simulink model "DJI_Mavic_Pro"  (R2022b)
settings: Solver=VariableStepAuto  StartTime=0.0  StopTime=100  RelTol=1e-3
libraries: slpidlib x3
settings Model: Creator=vikram  LastModifiedBy=vikram

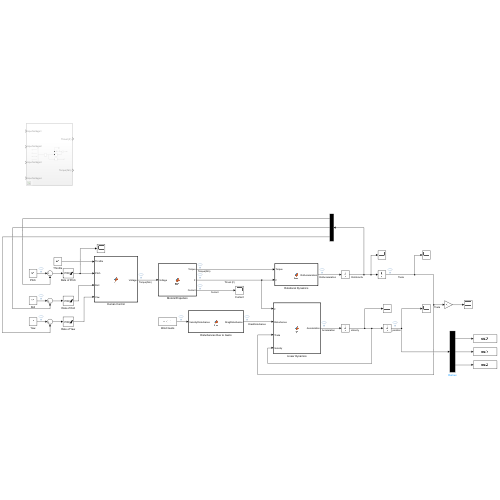
[thumbnail: Simulink's stored preview of the top-level diagram]
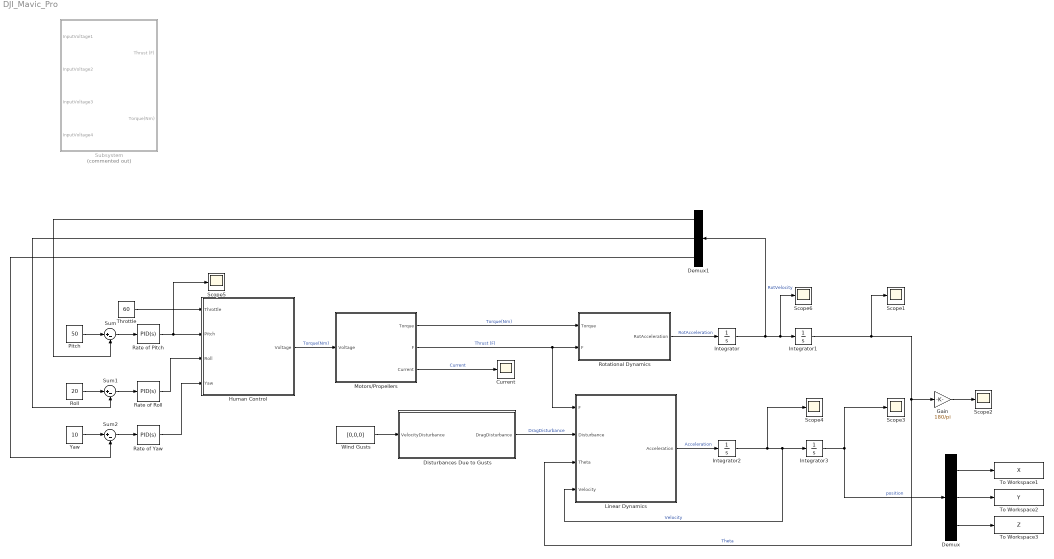
== system DJI_Mavic_Pro ==
  Current : Scope
  Demux : Demux  Outputs=3
  Demux1 : Demux  Outputs=3
  Disturbances Due to Gusts : MATLAB Function  TreatAsAtomicUnit=on
  Gain : Gain  Gain=180/pi
  Human Control : MATLAB Function  TreatAsAtomicUnit=on
  Integrator{,1..3} (4 alike) : Integrator
  Linear Dynamics : MATLAB Function  TreatAsAtomicUnit=on
  Motors/Propellers : MATLAB Function  TreatAsAtomicUnit=on
  Pitch : Constant  Value=50
  Rate of Pitch : slpidlib/PID Controller  Controller=PID  Form=Parallel  TimeDomain=Continuous-time  UseExternalTs=off  SampleTime=-1  IntegratorMethod=Forward Euler  FilterMethod=Forward Euler  ControllerParametersSource=internal  P=10  I=5  UseKiTs=off  D=0  N=100  UseFilter=on  TunerSelectOption=Transfer Function Based (PID Tuner App)  InitialConditionSource=internal  InitialConditionForIntegrator=0  InitialConditionForFilter=0  DifferentiatorICPrevScaledInput=0  ExternalReset=none  TrackingMode=off  Kt=1  LimitOutput=on  SatLimitsSource=internal  UpperSaturationLimit=100  LowerSaturationLimit=0  LinearizeAsGain=on  AntiWindupMode=clamping  Kb=1  LimitIntegrator=off  UpperIntegratorSaturationLimit=inf  LowerIntegratorSaturationLimit=-inf  POutMin=[]  POutMax=[]  IOutMin=[]  IOutMax=[]  DOutMin=[]  DOutMax=[]  NOutMin=[]  NOutMax=[]  SumOutMin=[]  SumOutMax=[]  SaturationOutMin=[]  SaturationOutMax=[]  PParamMin=[]  PParamMax=[]  IParamMin=[]  IParamMax=[]  DParamMin=[]  DParamMax=[]  NParamMin=[]  NParamMax=[]  KbParamMin=[]  KbParamMax=[]  KtParamMin=[]  KtParamMax=[]  KbOutMin=[]  KbOutMax=[]  KtOutMin=[]  KtOutMax=[]  IntegratorOutMin=[]  IntegratorOutMax=[]  FilterOutMin=[]  FilterOutMax=[]  SumI1OutMin=[]  SumI1OutMax=[]  SumI2OutMin=[]  SumI2OutMax=[]  SumI3OutMin=[]  SumI3OutMax=[]  SumI4OutMin=[]  SumI4OutMax=[]  SumDOutMin=[]  SumDOutMax=[]  DifferentiatorOutMin=[]  DifferentiatorOutMax=[]  FilterDiffOutCoefMin=[]  FilterDiffOutCoefMax=[]  ReciprocalOutMin=[]  ReciprocalOutMax=[]  SumDenOutMin=[]  SumDenOutMax=[]  SumNumOutMin=[]  SumNumOutMax=[]  DivideOutMin=[]  DivideOutMax=[]  UdiffTsProdOutMin=[]  UdiffTsProdOutMax=[]  NTsProdOutMin=[]  NTsProdOutMax=[]  UintegralTsProdOutMin=[]  UintegralTsProdOutMax=[]  UngainTsProdOutMin=[]  UngainTsProdOutMax=[]  ClampingZeroOutDataTypeStr=Inherit: Inherit via back propagation  ClampingZeroOutMin=[]  ClampingZeroOutMax=[]  FilterDenConstantOutDataTypeStr=Inherit: Inherit via back propagation  FilterDenConstantOutMin=[]  FilterDenConstantOutMax=[]  PCopyOutDataTypeStr=Inherit: Inherit via back propagation  PCopyOutMin=[]  PCopyOutMax=[]  NCopyOutDataTypeStr=Inherit: Inherit via back propagation  NCopyOutMin=[]  NCopyOutMax=[]  IntegratorContinuousStateAttributes=''  IntegratorStateMustResolveToSignalObject=off  IntegratorRTWStateStorageClass=Auto  FilterContinuousStateAttributes=''  FilterStateMustResolveToSignalObject=off  FilterRTWStateStorageClass=Auto  ParallelPVariant=InternalParameters  IdealPVariant=Disabled  IVariant=InternalParameters  DVariant=InternalParameters  IntegratorVariant=Continuous  SatVariant=Enabled  AWVariant=ContClampingParallel  PCopyVariant=Disabled  TRVariant=Disabled  FdbkBlocksVariant=Forward  IdealPFdbkVariant=Disabled  SatFdbkVariant=Disabled  DerivativeFilterVariant=ContFilter  NVariant=InternalParameters  NCopyVariant=Disabled  FilterICVariant=InternalICsFilter  IntegratorICVariant=InternalICs  ExternalResetVariant=Disabled  TRSumVariant=Passthrough  SumFdbkVariant=Disabled  SumVariant=Sum_PID  TsampFilterVariant=InternalTs  TsampNgainVariant=Passthrough  TsampIntegralVariant=Passthrough  ExternalSaturationOutDataTypeStr=Inherit: Same as second input
  Rate of Roll : slpidlib/PID Controller  Controller=PID  Form=Parallel  TimeDomain=Continuous-time  UseExternalTs=off  SampleTime=-1  IntegratorMethod=Forward Euler  FilterMethod=Forward Euler  ControllerParametersSource=internal  P=10  I=5  UseKiTs=off  D=0  N=100  UseFilter=on  TunerSelectOption=Transfer Function Based (PID Tuner App)  InitialConditionSource=internal  InitialConditionForIntegrator=0  InitialConditionForFilter=0  DifferentiatorICPrevScaledInput=0  ExternalReset=none  TrackingMode=off  Kt=1  LimitOutput=on  SatLimitsSource=internal  UpperSaturationLimit=100  LowerSaturationLimit=0  LinearizeAsGain=on  AntiWindupMode=clamping  Kb=1  LimitIntegrator=off  UpperIntegratorSaturationLimit=inf  LowerIntegratorSaturationLimit=-inf  POutMin=[]  POutMax=[]  IOutMin=[]  IOutMax=[]  DOutMin=[]  DOutMax=[]  NOutMin=[]  NOutMax=[]  SumOutMin=[]  SumOutMax=[]  SaturationOutMin=[]  SaturationOutMax=[]  PParamMin=[]  PParamMax=[]  IParamMin=[]  IParamMax=[]  DParamMin=[]  DParamMax=[]  NParamMin=[]  NParamMax=[]  KbParamMin=[]  KbParamMax=[]  KtParamMin=[]  KtParamMax=[]  KbOutMin=[]  KbOutMax=[]  KtOutMin=[]  KtOutMax=[]  IntegratorOutMin=[]  IntegratorOutMax=[]  FilterOutMin=[]  FilterOutMax=[]  SumI1OutMin=[]  SumI1OutMax=[]  SumI2OutMin=[]  SumI2OutMax=[]  SumI3OutMin=[]  SumI3OutMax=[]  SumI4OutMin=[]  SumI4OutMax=[]  SumDOutMin=[]  SumDOutMax=[]  DifferentiatorOutMin=[]  DifferentiatorOutMax=[]  FilterDiffOutCoefMin=[]  FilterDiffOutCoefMax=[]  ReciprocalOutMin=[]  ReciprocalOutMax=[]  SumDenOutMin=[]  SumDenOutMax=[]  SumNumOutMin=[]  SumNumOutMax=[]  DivideOutMin=[]  DivideOutMax=[]  UdiffTsProdOutMin=[]  UdiffTsProdOutMax=[]  NTsProdOutMin=[]  NTsProdOutMax=[]  UintegralTsProdOutMin=[]  UintegralTsProdOutMax=[]  UngainTsProdOutMin=[]  UngainTsProdOutMax=[]  ClampingZeroOutDataTypeStr=Inherit: Inherit via back propagation  ClampingZeroOutMin=[]  ClampingZeroOutMax=[]  FilterDenConstantOutDataTypeStr=Inherit: Inherit via back propagation  FilterDenConstantOutMin=[]  FilterDenConstantOutMax=[]  PCopyOutDataTypeStr=Inherit: Inherit via back propagation  PCopyOutMin=[]  PCopyOutMax=[]  NCopyOutDataTypeStr=Inherit: Inherit via back propagation  NCopyOutMin=[]  NCopyOutMax=[]  IntegratorContinuousStateAttributes=''  IntegratorStateMustResolveToSignalObject=off  IntegratorRTWStateStorageClass=Auto  FilterContinuousStateAttributes=''  FilterStateMustResolveToSignalObject=off  FilterRTWStateStorageClass=Auto  ParallelPVariant=InternalParameters  IdealPVariant=Disabled  IVariant=InternalParameters  DVariant=InternalParameters  IntegratorVariant=Continuous  SatVariant=Enabled  AWVariant=ContClampingParallel  PCopyVariant=Disabled  TRVariant=Disabled  FdbkBlocksVariant=Forward  IdealPFdbkVariant=Disabled  SatFdbkVariant=Disabled  DerivativeFilterVariant=ContFilter  NVariant=InternalParameters  NCopyVariant=Disabled  FilterICVariant=InternalICsFilter  IntegratorICVariant=InternalICs  ExternalResetVariant=Disabled  TRSumVariant=Passthrough  SumFdbkVariant=Disabled  SumVariant=Sum_PID  TsampFilterVariant=InternalTs  TsampNgainVariant=Passthrough  TsampIntegralVariant=Passthrough  ExternalSaturationOutDataTypeStr=Inherit: Same as second input
  Rate of Yaw : slpidlib/PID Controller  Controller=PID  Form=Parallel  TimeDomain=Continuous-time  UseExternalTs=off  SampleTime=-1  IntegratorMethod=Forward Euler  FilterMethod=Forward Euler  ControllerParametersSource=internal  P=10  I=5  UseKiTs=off  D=0  N=100  UseFilter=on  TunerSelectOption=Transfer Function Based (PID Tuner App)  InitialConditionSource=internal  InitialConditionForIntegrator=0  InitialConditionForFilter=0  DifferentiatorICPrevScaledInput=0  ExternalReset=none  TrackingMode=off  Kt=1  LimitOutput=on  SatLimitsSource=internal  UpperSaturationLimit=100  LowerSaturationLimit=0  LinearizeAsGain=on  AntiWindupMode=clamping  Kb=1  LimitIntegrator=off  UpperIntegratorSaturationLimit=inf  LowerIntegratorSaturationLimit=-inf  POutMin=[]  POutMax=[]  IOutMin=[]  IOutMax=[]  DOutMin=[]  DOutMax=[]  NOutMin=[]  NOutMax=[]  SumOutMin=[]  SumOutMax=[]  SaturationOutMin=[]  SaturationOutMax=[]  PParamMin=[]  PParamMax=[]  IParamMin=[]  IParamMax=[]  DParamMin=[]  DParamMax=[]  NParamMin=[]  NParamMax=[]  KbParamMin=[]  KbParamMax=[]  KtParamMin=[]  KtParamMax=[]  KbOutMin=[]  KbOutMax=[]  KtOutMin=[]  KtOutMax=[]  IntegratorOutMin=[]  IntegratorOutMax=[]  FilterOutMin=[]  FilterOutMax=[]  SumI1OutMin=[]  SumI1OutMax=[]  SumI2OutMin=[]  SumI2OutMax=[]  SumI3OutMin=[]  SumI3OutMax=[]  SumI4OutMin=[]  SumI4OutMax=[]  SumDOutMin=[]  SumDOutMax=[]  DifferentiatorOutMin=[]  DifferentiatorOutMax=[]  FilterDiffOutCoefMin=[]  FilterDiffOutCoefMax=[]  ReciprocalOutMin=[]  ReciprocalOutMax=[]  SumDenOutMin=[]  SumDenOutMax=[]  SumNumOutMin=[]  SumNumOutMax=[]  DivideOutMin=[]  DivideOutMax=[]  UdiffTsProdOutMin=[]  UdiffTsProdOutMax=[]  NTsProdOutMin=[]  NTsProdOutMax=[]  UintegralTsProdOutMin=[]  UintegralTsProdOutMax=[]  UngainTsProdOutMin=[]  UngainTsProdOutMax=[]  ClampingZeroOutDataTypeStr=Inherit: Inherit via back propagation  ClampingZeroOutMin=[]  ClampingZeroOutMax=[]  FilterDenConstantOutDataTypeStr=Inherit: Inherit via back propagation  FilterDenConstantOutMin=[]  FilterDenConstantOutMax=[]  PCopyOutDataTypeStr=Inherit: Inherit via back propagation  PCopyOutMin=[]  PCopyOutMax=[]  NCopyOutDataTypeStr=Inherit: Inherit via back propagation  NCopyOutMin=[]  NCopyOutMax=[]  IntegratorContinuousStateAttributes=''  IntegratorStateMustResolveToSignalObject=off  IntegratorRTWStateStorageClass=Auto  FilterContinuousStateAttributes=''  FilterStateMustResolveToSignalObject=off  FilterRTWStateStorageClass=Auto  ParallelPVariant=InternalParameters  IdealPVariant=Disabled  IVariant=InternalParameters  DVariant=InternalParameters  IntegratorVariant=Continuous  SatVariant=Enabled  AWVariant=ContClampingParallel  PCopyVariant=Disabled  TRVariant=Disabled  FdbkBlocksVariant=Forward  IdealPFdbkVariant=Disabled  SatFdbkVariant=Disabled  DerivativeFilterVariant=ContFilter  NVariant=InternalParameters  NCopyVariant=Disabled  FilterICVariant=InternalICsFilter  IntegratorICVariant=InternalICs  ExternalResetVariant=Disabled  TRSumVariant=Passthrough  SumFdbkVariant=Disabled  SumVariant=Sum_PID  TsampFilterVariant=InternalTs  TsampNgainVariant=Passthrough  TsampIntegralVariant=Passthrough  ExternalSaturationOutDataTypeStr=Inherit: Same as second input
  Roll : Constant  Value=20
  Rotational Dynamics : MATLAB Function  TreatAsAtomicUnit=on
  Scope{1..6} (6 alike) : Scope
  Subsystem : Subsystem  Commented=on
  Sum : Sum  Inputs=|+-
  Sum1 : Sum  Inputs=|+-
  Sum2 : Sum  Inputs=|+-
  Throttle : Constant  Value=60
  To Workspace1 : ToWorkspace  VariableName=X  SampleTime=-1
      settings: Save2DSignal=2-D array (concatenate along first dimension)
  To Workspace2 : ToWorkspace  VariableName=Y  SampleTime=-1
      settings: Save2DSignal=2-D array (concatenate along first dimension)
  To Workspace3 : ToWorkspace  VariableName=Z  SampleTime=-1
      settings: Save2DSignal=2-D array (concatenate along first dimension)
  Wind Gusts : Constant  Value=[0,0,0]
  Yaw : Constant  Value=10
  wires:
  Motors/Propellers/2(F) -> Linear Dynamics/1(F), Rotational Dynamics/2(F)  "Thrust (F)"
  Motors/Propellers/3(Current) -> Current/1  "Current"
  Motors/Propellers/1(Torque) -> Rotational Dynamics/1(Torque)  "Torque(Nm)"
  Integrator/1 -> Demux1/1, Scope6/1, Integrator1/1  "RotVelocity"
  Rotational Dynamics/1(RotAcceleration) -> Integrator/1  "RotAcceleration"
  Integrator1/1 -> Gain/1, Linear Dynamics/3(Theta), Scope1/1  "Theta"
  Linear Dynamics/1(Acceleration) -> Integrator2/1  "Acceleration"
  Integrator2/1 -> Scope4/1, Linear Dynamics/4(Velocity), Integrator3/1  "Velocity"
  Integrator3/1 -> Demux/1, Scope3/1  "position"
  Human Control/1(Voltage) -> Motors/Propellers/1(Voltage)  "Torque(Nm)"
  Pitch/1 -> Sum/1
  Throttle/1 -> Human Control/1(Throttle)
  Wind Gusts/1 -> Disturbances Due to Gusts/1(VelocityDisturbance)
  Disturbances Due to Gusts/1(DragDisturbance) -> Linear Dynamics/2(Disturbance)  "DragDisturbance"
  Gain/1 -> Scope2/1
  Demux/3 -> To Workspace3/1
  Demux/2 -> To Workspace2/1
  Rate of Pitch/1 -> Scope5/1, Human Control/2(Pitch)
  Sum/1 -> Rate of Pitch/1
  Demux/1 -> To Workspace1/1
  Demux1/1 -> Sum/2
  Sum1/1 -> Rate of Roll/1
  Roll/1 -> Sum1/1
  Rate of Roll/1 -> Human Control/3(Roll)
  Demux1/2 -> Sum1/2
  Yaw/1 -> Sum2/1
  Sum2/1 -> Rate of Yaw/1
  Rate of Yaw/1 -> Human Control/4(Yaw)
  Demux1/3 -> Sum2/2

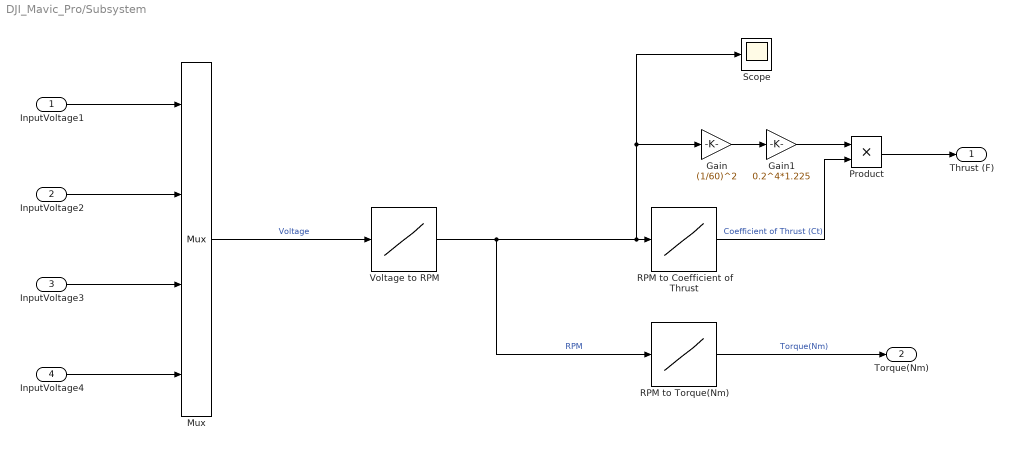
== system DJI_Mavic_Pro/Subsystem ==
  InputVoltage1 : Inport
  InputVoltage2 : Inport  Port=2
  InputVoltage3 : Inport  Port=3
  InputVoltage4 : Inport  Port=4
  " RPM to Torque(Nm)" : Lookup_n-D  NumberOfTableDimensions=1  BreakpointsForDimension1=|  Table=|  InternalRulePriority=Speed  RndMeth=Simplest
      BreakpointsForDimension1=|
      | [1000
      | 2000
      | 3000
      | 4000
      | 5000
      | 6000
      | 7000
      | 8000
      | 9000
      | 10000
      | 11000
      | 12000
      | 13000
      | 13999
      | 15000
      | 16000
      | 17000
      | 18000
      | 19000
      | 20000
      | 21000
      | 22000
      | 23000
      | 24000
      | 25000
      | 26000
      | 26999
      | 29000
      | 30000]
      Table=|
      | [0.000790893803
      | 0.003050590383
      | 0.00677908974
      | 0.01220236153
      | 0.0190944361
      | 0.02745531345
      | 0.03751096323
      | 0.04926138544
      | 0.06157673181
      | 0.07524789611
      | 0.09027487837
      | 0.1067706634
      | 0.1246222664
      | 0.1485750501
      | 0.1842782561
      | 0.2258566732
      | 0.2743271648
      | 0.3309325641
      | 0.3974806284
      | 0.4765700087
      | 0.5719292044
      | 0.6912411838
      | 0.868853335
      | 1.456374446
      | 1.887185599
      | 1.880745464
      | 2.452787653
      | 2.724629151
      | 2.137108041]
  Gain : Gain  Gain=(1/60)^2
  Gain1 : Gain  Gain=0.2^4*1.225
  Mux : Mux
  Product : Product
  RPM to Coefficient of Thrust : Lookup_n-D  NumberOfTableDimensions=1  BreakpointsForDimension1=|  Table=|  InternalRulePriority=Speed  RndMeth=Simplest
      BreakpointsForDimension1=|
      | [1000
      | 2000
      | 3000
      | 4000
      | 5000
      | 6000
      | 7000
      | 8000
      | 9000
      | 10000
      | 11000
      | 12000
      | 13000
      | 13999
      | 15000
      | 16000
      | 17000
      | 18000
      | 19000
      | 20000
      | 21000
      | 22000
      | 23000
      | 24000
      | 25000
      | 26000
      | 26999
      | 29000
      | 30000]
      Table=|
      | [0.1017
      | 0.1018
      | 0.1018
      | 0.102
      | 0.1021
      | 0.1023
      | 0.1025
      | 0.1027
      | 0.1028
      | 0.103
      | 0.1033
      | 0.1037
      | 0.1041
      | 0.1047
      | 0.1056
      | 0.1065
      | 0.1074
      | 0.1084
      | 0.1094
      | 0.1104
      | 0.1115
      | 0.1128
      | 0.1147
      | 0.1177
      | 0.1194
      | 0.1188
      | 0.12
      | 0.1167
      | 0.1113]
  Scope : Scope
  Voltage to RPM : Lookup_n-D  NumberOfTableDimensions=1  BreakpointsForDimension1="[0\t0.570000000000000\t1.14000000000000\t1.71000000000000\t2.28000000000000\t2.85000000000000\t3.42000000000000\t3.99000000000000\t4.56000000000000\t5.13000000000000\t5.70000000000000\t6.27000000000000\t6.84000000000000\t7.41000000000000\t7.98000000000000\t8.55000000000000\t9.12000000000000\t9.69000000000000\t10.2600000000000\t10.8300000000000\t11.4000000000000]"  Table="[0\t797.501250000000\t1592.01000000000\t2380.53375000000\t3160.08000000000\t3927.65625000000\t4680.27000000000\t5414.92875000000\t6128.64000000000\t6818.41125000000\t7481.25000000000\t8114.16375000000\t8714.16000000000\t9278.24625000000\t9803.43000000000\t10286.7187500000\t10725.1200000000\t11115.6412500000\t11455.2900000000\t11741.0737500000\t11970]"  InternalRulePriority=Speed  RndMeth=Simplest
  Thrust (F) : Outport
  Torque(Nm) : Outport  Port=2
  wires:
  RPM to Coefficient of Thrust/1 -> Product/2  "Coefficient of Thrust (Ct)"
  Voltage to RPM/1 -> Gain/1, Scope/1, RPM to Coefficient of Thrust/1, " RPM to Torque(Nm)"/1  "RPM"
  " RPM to Torque(Nm)"/1 -> Torque(Nm)/1  "Torque(Nm)"
  Mux/1 -> Voltage to RPM/1  "Voltage"
  InputVoltage1/1 -> Mux/1
  InputVoltage2/1 -> Mux/2
  InputVoltage4/1 -> Mux/4
  InputVoltage3/1 -> Mux/3
  Gain1/1 -> Product/1
  Gain/1 -> Gain1/1
  Product/1 -> Thrust (F)/1

== matlab function DJI_Mavic_Pro/Rotational Dynamics ==
  data: Torque input; RotAcceleration output; F input
function RotAcceleration = fcn(Torque,F)
Moment=[0 0 0];
RotAcceleration=[0 0 0];
I=[0.003,0.003,0.007];
Moment(1)=(F(3)+F(4))*0.237/2-(F(1)+F(2))*0.237/2;
Moment(2)=(F(3)+F(2))*0.237/2-(F(1)+F(4))*0.237/2;
Moment(3)=Torque(4)-Torque(1)+Torque(2)-Torque(3);

for i=1:3
    RotAcceleration(i)=Moment(i)/I(i);
end

== matlab function DJI_Mavic_Pro/Motors//Propellers ==
  data: Voltage input; Torque output; F output; Current output
function [Torque, F, Current] = fcn(Voltage)

RPM = [0 0 0 0];
Torque = [0 0 0 0];
Current = [0 0 0 0];
F = [0 0 0 0];

for i=1:4
    RPM(i)=-2.6931*Voltage(i)^3+1400*Voltage(i);
    Ct= 2*10^-15*RPM(i)^3-4*10^-11*RPM(i)^2+3*10^-7*RPM(i)+0.1013;
    F(i)= Ct*1.225*(RPM(i)/60)^2*0.2^4;
    Torque(i)= 4*10^-14*RPM(i)^3+8*10^-12*RPM(i)^2+3*10^-6*RPM(i);
    Current(i)= 1400*Torque(i);
end

== matlab function DJI_Mavic_Pro/Linear Dynamics ==
  data: F input; Disturbance input; Acceleration output; Theta input; Velocity input
function Acceleration = fcn(F,Disturbance,Theta,Velocity)
m=0.743;
g=9.81;
A=[0.0197 0.0197 0.0512];
rho=1.225;
Cd=1;

Acceleration=[0 0 0];
Force=[0 0 0];
Fprop=[0 0 0];

Fprop(1)=sin(Theta(2))*cos(Theta(1))*(F(1)+F(2)+F(3)+F(4));
Fprop(2)=sin(Theta(1))*cos(Theta(2))*(F(1)+F(2)+F(3)+F(4));
Fprop(3)=cos(Theta(1))*cos(Theta(2))*(F(1)+F(2)+F(3)+F(4));

ThetaXY=-atan2(Fprop(1),Fprop(2));
XY2D=sqrt(Fprop(1)^2+Fprop(2)^2);

if Fprop(3)>=0
	Fprop(1)=XY2D*sin(Theta(3)+ThetaXY);
	Fprop(2)=XY2D*cos(Theta(3)+ThetaXY);
else
	Fprop(1)=XY2D*sin(-Theta(3)+ThetaXY);
	Fprop(2)=XY2D*cos(-Theta(3)+ThetaXY);
end

if Velocity(1)<0
	Force(1)=Fprop(1)-Disturbance(1)+0.5*rho*Velocity(1)^2*A(1)*Cd;
else
	Force(1)=Fprop(1)-Disturbance(1)-0.5*rho*Velocity(1)^2*A(1)*Cd;
end

if Velocity(2)<0
	Force(2)=Fprop(2)-Disturbance(2)+0.5*rho*Velocity(2)^2*A(2)*Cd;
else
	Force(2)=Fprop(2)-Disturbance(2)-0.5*rho*Velocity(2)^2*A(2)*Cd;
end

if Velocity(3)<0
	Force(3)=Fprop(3)-Disturbance(3)+0.5*rho*Velocity(3)^2*A(3)*Cd-m*g;
else
	Force(3)=Fprop(3)-Disturbance(3)-0.5*rho*Velocity(3)^2*A(3)*Cd-m*g;
end

for i=1:3
	Acceleration(i)=Force(i)/m;
end

== matlab function DJI_Mavic_Pro/Human Control ==
  data: Throttle input; Voltage output; Pitch input; Roll input; Yaw input
function Voltage = fcn(Throttle,Pitch,Roll,Yaw)
Correct=0;
if (Pitch/2+Roll/2+Yaw/2)>(100-Throttle)
	Correct=((Pitch/2+Roll/2+Yaw/2)-(100-Throttle));
end
if(Pitch/2+Roll/2+Yaw/2)>(Throttle)
	if Correct<((Pitch/2+Roll/2+Yaw/2)-(Throttle))
	   Correct=((Pitch/2+Roll/2+Yaw/2)-(Throttle));
	end
end

if Correct~=0
Pitch=Pitch-Correct/3*2;
Roll=Roll-Correct/3*2;
end

Voltage=[(Throttle-Pitch/2-Roll/2-Yaw/2)*11.4/100
	(Throttle-Pitch/2+Roll/2+Yaw/2)*11.4/100
	(Throttle+Pitch/2+Roll/2-Yaw/2)*11.4/100
	(Throttle+Pitch/2-Roll/2+Yaw/2)*11.4/100];

== matlab function DJI_Mavic_Pro/Disturbances Due to Gusts ==
  data: VelocityDisturbance input; DragDisturbance output
function DragDisturbance = fcn(VelocityDisturbance)
A=[0.0197 0.0197 0.0197*2*1.3];
DragDisturbance=[0 0 0];
rho=1.225;
Cd=1;

for i=1:3
	if VelocityDisturbance(i)<0
		DragDisturbance(i)=0.5*rho*VelocityDisturbance(i)^2*A(i)*Cd;
	else
		DragDisturbance(i)=-0.5*rho*VelocityDisturbance(i)^2*A(i)*Cd;
	end
end
